simulink model "AVR"  (R2016a)
settings: Solver=VariableStepAuto  StartTime=0.0  StopTime=10.0  RelTol=1e-3
settings Model: Creator=EBUKA  LastModifiedBy=EBUKA
settings GRTTargetCC: GeneratePreprocessorConditionals=Use local settings

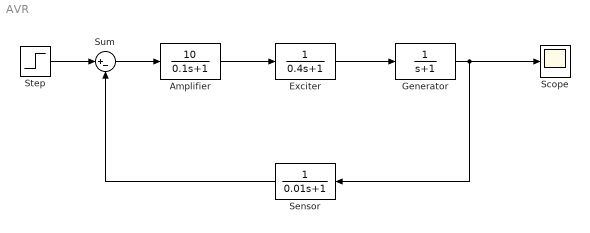
== system AVR ==
  Amplifier : TransferFcn  Numerator=[10]  Denominator=[0.1 1]
  Exciter : TransferFcn  Denominator=[0.4 1]
  Generator : TransferFcn  Denominator=[1 1]
  Scope : Scope
  Sensor : TransferFcn  Denominator=[0.01 1]
  Step : Step  SampleTime=0
  Sum : Sum  Inputs=|+-
  wires:
  Exciter/1 -> Generator/1
  Amplifier/1 -> Exciter/1
  Generator/1 -> Scope/1, Sensor/1
  Sum/1 -> Amplifier/1
  Sensor/1 -> Sum/2
  Step/1 -> Sum/1
